simulink model "Inverted_Pendulum_control"  (R2024a)
settings: Solver=VariableStepAuto  StartTime=0.0  StopTime=10.0  RelTol=1e-3
libraries: fuzblock x1
settings Model: Creator=Miko  LastModifiedBy=Miko

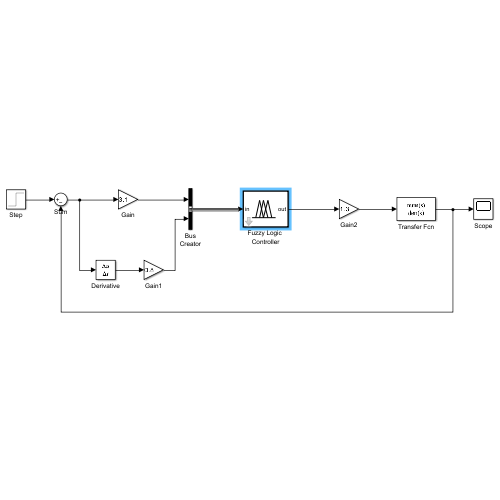
[thumbnail: Simulink's stored preview of the top-level diagram]
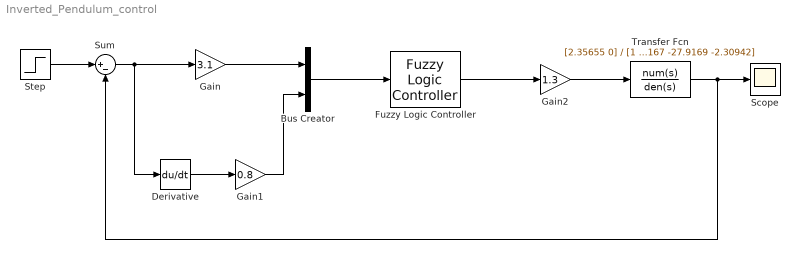
== system Inverted_Pendulum_control ==
  Bus Creator : BusCreator  Inputs=2
  Derivative : Derivative
  Fuzzy Logic Controller : fuzblock/Fuzzy Logic  Controller  FIS='ipFIS.fis'  OutputSampleNumber=101  DataType=double  FuzzifiedInputs=off  RuleFiringStrengths=off  RuleOutputs=off  AggregatedOutputs=off  SimulateUsing=Interpreted execution  OutOfRangeInputValueMessage=warning  NoRuleFiredMessage=warning  EmptyOutputFuzzySetMessage=warning
  Gain : Gain  Gain=3.1
  Gain1 : Gain  Gain=0.8
  Gain2 : Gain  Gain=1.3
  Scope : Scope
  Step : Step  SampleTime=0
  Sum : Sum  Inputs=|+-
  Transfer Fcn : TransferFcn  Numerator=[2.35655 0]  Denominator=[1 0.0883167 -27.9169 -2.30942]
  wires:
  Step/1 -> Sum/1
  Sum/1 -> Derivative/1, Gain/1
  Bus Creator/1 -> Fuzzy Logic Controller/1
  Gain/1 -> Bus Creator/1
  Derivative/1 -> Gain1/1
  Gain1/1 -> Bus Creator/2
  Fuzzy Logic Controller/1 -> Gain2/1
  Gain2/1 -> Transfer Fcn/1
  Transfer Fcn/1 -> Sum/2, Scope/1
